simulink model "virtualPendulumModel"  (R2022a)
settings: Solver=FixedStepAuto  StartTime=0.0  StopTime=10  FixedStep=model.ts  RelTol=1e-3
InitFcn:
  | Ts = 0.01;
undefined symbols (not defined in the file): Discrete, model, Time, X, Y, Z
libraries: sm_lib x8, nesl_utility x3, simulink x2, sharedTrackingLibrary x1, ctrlSharedLib x1
settings Model: Creator=mulusoy  LastModifiedBy=gioel
settings DebuggingCC: UnconnectedInputMsg=warning  UnconnectedOutputMsg=warning  UnconnectedLineMsg=warning
settings RTWCC: DLArmComputeVersion=19.05
settings ExplorerConfigSet: InternalSimMechanicsExplorerSettings="<ExplorerConfiguration><canonicalview>planar_xy</canonicalview><AnimationSetting><BasePlaybackSpeed>1.0</BasePlaybackSpeed><PlaybackSpeedFactor>1.0</PlaybackSpeedFactor></AnimationSetting><TilePanel><TileInfo><Tiles Columns=\"1\" Count=\"1\" Rows=\"1\"><Column Weight=\"1\"/><Row Weight=\"1\"/><Tile Height=\"1\" Width=\"1\" X=\"0\" Y=\"0\"/></Tiles></TileInfo><SceneInfo><SceneViewer><BGColor><R>0.60000002384185791</R><G>0.60000002384185791</G><B>0.60000002384185791</B></BGColor><Camera><DoPerspective>off</DoPerspective><Position><X>-2.81337411700555151e-09</X><Y>-0.263610325606282447</Y><Z>1.00000001491760937</Z></Position><Center><X>-2.81337411700555151e-09</X><Y>-0.263610325606282447</Y><Z>1.49176093700020829e-08</Z></Center><Up><X>0</X><Y>1</Y><Z>0</Z></Up><ViewLimDist>1</ViewLimDist><YLim>0.297268618643283855</YLim><XLim>0.57836459223084502</XLim></Camera></SceneViewer></SceneInfo></TilePanel><MechEditorPanel><Cameras/><GfxPanelCameraMap/><VideoCreator><PlaybackSpeedRatio>1.0</PlaybackSpeedRatio><FrameRate>30</FrameRate><VideoFormat>Motion JPEG AVI</VideoFormat><FrameSize>auto</FrameSize></VideoCreator></MechEditorPanel></ExplorerConfiguration>"

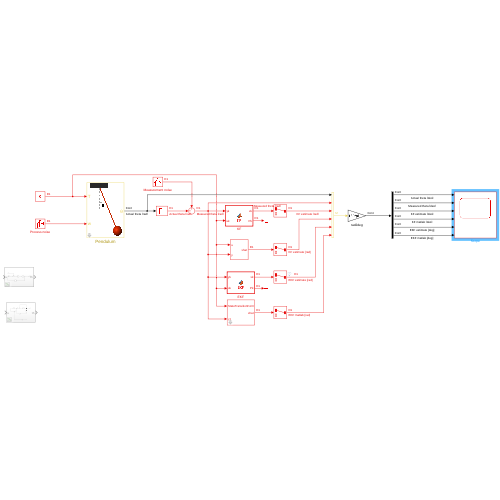
[thumbnail: Simulink's stored preview of the top-level diagram]
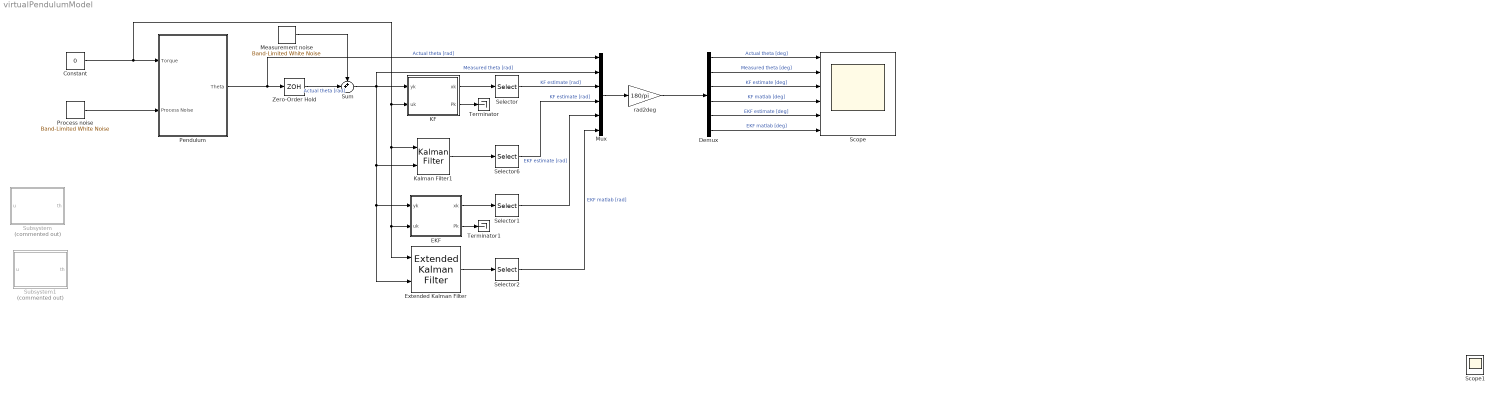
== system virtualPendulumModel ==
  Constant : Constant  Value=0  SampleTime=model.ts
  Demux : Demux  Outputs=6
  EKF : MATLAB Function  TreatAsAtomicUnit=on
  Extended Kalman Filter : sharedTrackingLibrary/Extended Kalman Filter  StateTransitionFcn=myStateTransitionFcn  HasStateTransitionJacobianFcn=off  HasAdditiveProcessNoise=Additive  ProcessNoise=model.Q  HasTimeVaryingProcessNoise=off  HasStateTransitionFcnExtraArgument=1  InitialState=[model.theta0; model.theta_dot0]  InitialStateCovariance=model.dis_lin.P0  MeasurementFcn1=myMeasurementFcn  HasMeasurementJacobianFcn1=off  HasMeasurementEnablePort1=off  HasAdditiveMeasurementNoise1=Additive  MeasurementNoise1=model.R  HasTimeVaryingMeasurementNoise1=off  HasMeasurementFcnExtraArgument1=0  HasMeasurementWrapping1=off  MeasurementFcn2=myMeasurementFcn  HasMeasurementJacobianFcn2=off  HasMeasurementEnablePort2=off  HasAdditiveMeasurementNoise2=Additive  MeasurementNoise2=1  HasTimeVaryingMeasurementNoise2=off  HasMeasurementFcnExtraArgument2=0  HasMeasurementWrapping2=off  MeasurementFcn3=myMeasurementFcn  HasMeasurementJacobianFcn3=off  HasMeasurementEnablePort3=off  HasAdditiveMeasurementNoise3=Additive  MeasurementNoise3=1  HasTimeVaryingMeasurementNoise3=off  HasMeasurementFcnExtraArgument3=0  HasMeasurementWrapping3=off  MeasurementFcn4=myMeasurementFcn  HasMeasurementJacobianFcn4=off  HasMeasurementEnablePort4=off  HasAdditiveMeasurementNoise4=Additive  MeasurementNoise4=1  HasTimeVaryingMeasurementNoise4=off  HasMeasurementFcnExtraArgument4=0  HasMeasurementWrapping4=off  MeasurementFcn5=myMeasurementFcn  HasMeasurementJacobianFcn5=off  HasMeasurementEnablePort5=off  HasAdditiveMeasurementNoise5=Additive  MeasurementNoise5=1  HasTimeVaryingMeasurementNoise5=off  HasMeasurementFcnExtraArgument5=0  HasMeasurementWrapping5=off  EnableMultirate=off  StateTransitionFcnSampleTime=1  MeasurementFcn1SampleTime=1  MeasurementFcn2SampleTime=1  MeasurementFcn3SampleTime=1  MeasurementFcn4SampleTime=1  MeasurementFcn5SampleTime=1  UseCurrentEstimator=on  OutputStateCovariance=off  DataType=double  SampleTime=model.ts  NumberOfMeasurements=1
      settings: SourceProductBaseCode=TF,AE,PW,CT,DR,ID,LP,NV,AR,RO,RR,UV,VE
  KF : MATLAB Function  TreatAsAtomicUnit=on
  Kalman Filter1 : ctrlSharedLib/Kalman Filter  TimeDomain=Discrete-Time  UseCurrentEstimator=on  ModelSource=Individual A, B, C, D matrices  ModelSourceVariable=ss(0.95,1,1,0,1)  A=model.dis_lin.A  B=model.dis_lin.B  C=model.dis_lin.C  D=model.dis_lin.D  NumberOfStates=1  NumberOfInputs=1  NumberOfOutputs=1  InitialEstimateSource=Dialog  X0=[model.theta0; model.theta_dot0]  P0=10  UseK=off  UseGH=off  NumberOfProcessNoiseInputs=1  G=1  TimeInvariantG=on  H=0  TimeInvariantH=on  Q=model.Q  TimeInvariantQ=on  R=model.R  TimeInvariantR=on  N=0  TimeInvariantN=on  AddInputPort=on  AddEnablePort=off  OutputEstimatedY=off  OutputP=off  Ts=model.ts
  Measurement noise : simulink/Sources/Band-Limited White Noise  Cov=model.R*model.ts  Ts=model.ts  seed=[23341]
  Mux : Mux  Inputs=6
  Pendulum : Subsystem  mask{theta_0=model.theta0, theta_dot_0=model.theta_dot0}
      mask prompts: theta_0 "Initial value of theta"; theta_dot_0 "Initial value of theta_dot"
      mask Display:
      | image('pend.png');
      | port_label('input',1,'T');
      | port_label('input',2,'w');
      | port_label('output',1,'\theta','interpreter','tex');
  Process noise : simulink/Sources/Band-Limited White Noise  Cov=model.Q(2,2)*model.ts  Ts=model.ts  seed=[23341]
  Scope : Scope  NumInputPorts=6
  Selector{,1..2,6} (4 alike) : Selector  InputPortWidth=2  IndexOptions=Index vector (dialog)  Indices=[1]  OutputSizes=1
  Subsystem : Subsystem  Commented=on
  Subsystem1 : Subsystem  Commented=on
  Sum : Sum  Inputs=++|
  Terminator : Terminator
  Terminator1 : Terminator
  Zero-Order Hold : ZeroOrderHold  SampleTime=model.ts
  rad2deg : Gain  Gain=180/pi
  Scope1 : Scope
  wires:
  Measurement noise/1 -> Sum/1
  Process noise/1 -> Pendulum/2(Process Noise)
  KF/1(xk) -> Selector/1
  Selector/1 -> Mux/3  "KF estimate [rad]"
  Mux/1 -> rad2deg/1
  KF/2(Pk) -> Terminator/1
  Sum/1 -> Extended Kalman Filter/2, EKF/1(yk), Kalman Filter1/2, Mux/2, KF/1(yk)  "Measured theta [rad]"
  Zero-Order Hold/1 -> Sum/2  "Actual theta [rad]"
  Pendulum/1(Theta) -> Mux/1, Zero-Order Hold/1  "Actual theta [rad]"
  EKF/2(Pk) -> Terminator1/1
  EKF/1(xk) -> Selector1/1
  Selector1/1 -> Mux/5  "EKF estimate [rad]"
  Constant/1 -> EKF/2(uk), Extended Kalman Filter/1, Kalman Filter1/1, KF/2(uk), Pendulum/1(Torque)
  Extended Kalman Filter/1 -> Selector2/1
  Selector2/1 -> Mux/6  "EKF matlab [rad]"
  Kalman Filter1/1 -> Selector6/1
  Demux/6 -> Scope/6  "EKF matlab [deg]"
  Demux/5 -> Scope/5  "EKF estimate [deg]"
  Demux/3 -> Scope/3  "KF estimate [deg]"
  Demux/2 -> Scope/2  "Measured theta [deg]"
  Demux/1 -> Scope/1  "Actual theta [deg]"
  rad2deg/1 -> Demux/1
  Selector6/1 -> Mux/4  "KF estimate [rad]"
  Demux/4 -> Scope/4  "KF matlab [deg]"

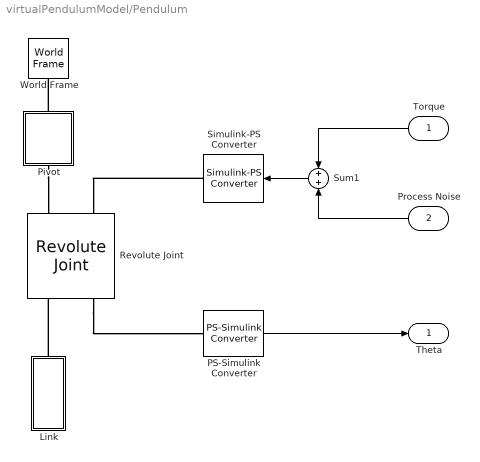
== system virtualPendulumModel/Pendulum ==
  Torque : Inport
  Process Noise : Inport  Port=2
  Link : Subsystem  Tag=CustomStyle
  PS-Simulink Converter : nesl_utility/PS-Simulink Converter  PhysicalDomain=network_engine_domain  SubClassName=ps_output  LeftPortType=input  RightPortType=output  PseudoPeriodic=off  Frequencies=[]  VectorFormat=1-D array  Unit=1  AffineConversion=off
      settings: SourceProductBaseCode=SS,PW,VE
  Pivot : Subsystem  Tag=CustomStyle
  Revolute Joint : sm_lib/Joints/Revolute Joint  JointMode=Normal  SenseConstraintForce=off  SenseConstraintForceX=off  SenseConstraintForceY=off  SenseConstraintForceZ=off  SenseConstraintTorque=off  SenseConstraintTorqueX=off  SenseConstraintTorqueY=off  SenseConstraintTorqueZ=off  SenseTotalForce=off  SenseTotalForceX=off  SenseTotalForceY=off  SenseTotalForceZ=off  SenseTotalTorque=off  SenseTotalTorqueX=off  SenseTotalTorqueY=off  SenseTotalTorqueZ=off  CompositeWrenchDir=FollowerOnBase  CompositeWrenchFrame=BaseFrame  EquilibriumPosition=0  EquilibriumPositionUnits=rad  SpringStiffness=0  SpringStiffnessUnits=N*m/rad  DampingCoefficient=0  DampingCoefficientUnits=N*m/(rad/s)  TorqueActuationMode=InputTorque  MotionActuationMode=ComputedMotion  SensePosition=on  SenseVelocity=off  SenseAcceleration=off  SenseTorqueForce=off  SenseLowerLimitTorqueForce=off  SenseUpperLimitTorqueForce=off  LowerLimitSpecify=off  LowerLimitBound=-90  LowerLimitBoundUnits=deg  LowerLimitStiffness=1e4  LowerLimitStiffnessUnits=N*m/deg  LowerLimitDamping=10  LowerLimitDampingUnits=N*m/(deg/s)  LowerLimitTransitionRegionWidth=0.1  LowerLimitTransitionRegionWidthUnits=deg  UpperLimitSpecify=off  UpperLimitBound=90  UpperLimitBoundUnits=deg  UpperLimitStiffness=1e4  UpperLimitStiffnessUnits=N*m/deg  UpperLimitDamping=10  UpperLimitDampingUnits=N*m/(deg/s)  UpperLimitTransitionRegionWidth=0.1  UpperLimitTransitionRegionWidthUnits=deg  PositionTargetSpecify=on  PositionTargetPriority=High  PositionTargetValue=model.theta0  PositionTargetValueUnits=rad  VelocityTargetSpecify=on  VelocityTargetPriority=High  VelocityTargetValue=model.theta_dot0  VelocityTargetValueUnits=rad/s
  Simulink-PS Converter : nesl_utility/Simulink-PS Converter  PhysicalDomain=network_engine_domain  SubClassName=ps_input  LeftPortType=input  RightPortType=output  PseudoPeriodic=off  Frequencies=[]  NoiseDistribution=none  NoiseParameters=[]  Unit=1  AffineConversion=off  FilteringAndDerivatives=provide  SimscapeFilterOrder=1  InputFilterTimeConstant=0.001  UdotUserProvided=0
      settings: SourceProductBaseCode=SS,PW,VE
  Sum1 : Sum  Inputs=+|+
  World Frame : sm_lib/Frames and Transforms/World Frame
  Theta : Outport
  wires:
  Sum1/1 -> Simulink-PS Converter/1
  Torque/1 -> Sum1/1
  Process Noise/1 -> Sum1/2
  PS-Simulink Converter/1 -> Theta/1
  connections:
  Pivot/LConn1 -- World Frame/RConn1
  Pivot/RConn1 -- Revolute Joint/LConn1
  Link/RConn1 -- Revolute Joint/RConn1
  Revolute Joint/RConn2 -- PS-Simulink Converter/LConn1
  Simulink-PS Converter/RConn1 -- Revolute Joint/LConn2

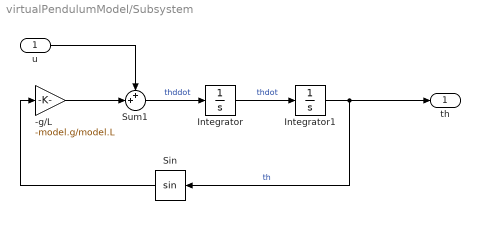
== system virtualPendulumModel/Subsystem ==
  u : Inport
  -g/L : Gain  Gain=-model.g/model.L
  Integrator : Integrator  InitialCondition=model.theta_dot0
  Integrator1 : Integrator  InitialCondition=model.theta0
  Sin : Trigonometry
  Sum1 : Sum  Inputs=++|
  th : Outport
  wires:
  Sum1/1 -> Integrator/1  "thddot"
  Integrator/1 -> Integrator1/1  "thdot"
  Sin/1 -> -g/L/1
  u/1 -> Sum1/1
  Integrator1/1 -> th/1, Sin/1  "th"
  -g/L/1 -> Sum1/2

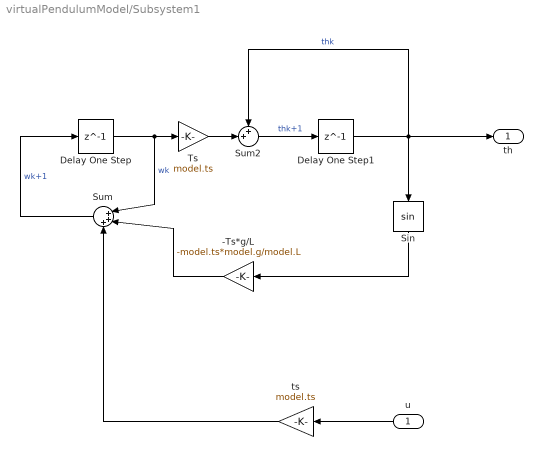
== system virtualPendulumModel/Subsystem1 ==
  u : Inport
  -Ts*g/L : Gain  Gain=-model.ts*model.g/model.L
  Delay One Step : Delay  DelayLength=1  InitialCondition=model.theta_dot0
  Delay One Step1 : Delay  DelayLength=1  InitialCondition=model.theta0
  Sin : Trigonometry
  Sum : Sum  Inputs=|+++
  Sum2 : Sum  Inputs=++|
  Ts : Gain  Gain=model.ts
  ts : Gain  Gain=model.ts
  th : Outport
  wires:
  -Ts*g/L/1 -> Sum/2
  ts/1 -> Sum/3
  u/1 -> ts/1
  Sin/1 -> -Ts*g/L/1
  Delay One Step/1 -> Sum/1, Ts/1  "wk"
  Ts/1 -> Sum2/2
  Sum2/1 -> Delay One Step1/1  "thk+1"
  Delay One Step1/1 -> th/1, Sin/1, Sum2/1  "thk"
  Sum/1 -> Delay One Step/1  "wk+1"

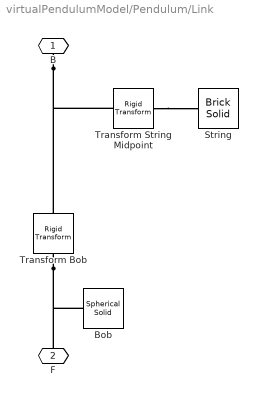
== system virtualPendulumModel/Pendulum/Link ==
  Bob : sm_lib/Body Elements/Spherical Solid  GraphicAmbientColor=[0.15 0.15 0.15 1.0]  BasedOnType=Density  CenterOfMass=[0 0 0]  CenterOfMassUnits=m  GraphicDiffuseColor=[1.0 0.2 0.0]  Density=1000  DensityUnits=kg/(m^3)  DoExposeReferenceFrame=on  GraphicEmissiveColor=[0.0 0.0 0.0 1.0]  ExportEntireGeometry=off  SerializedExposedGeometries=<ExposedGeometries/>  SerializedFrames=<Frames/>  MarkerShape=Sphere  MarkerSize=10  GraphicType=FromGeometry  InertiaType=PointMass  Mass=model.m  MassUnits=kg  MomentsOfInertia=[1 1 1]*1e-3  MomentsOfInertiaUnits=kg*m^2  GraphicOpacity=1.0  ProductsOfInertia=[0 0 0]  ProductsOfInertiaUnits=kg*m^2  GraphicShininess=75  GraphicSpecularColor=[0.5 0.5 0.5 1.0]  SphereRadius=0.05  SphereRadiusUnits=m  GraphicVisPropType=SimpleVisualProperties
  String : sm_lib/Body Elements/Brick Solid  GraphicAmbientColor=[0.15 0.15 0.15 1.0]  BasedOnType=Density  BrickDimensions=[0.01 model.L 0.01]  BrickDimensionUnits=m  CenterOfMass=[0 0 0]  CenterOfMassUnits=m  GraphicDiffuseColor=[1.0 0.2 0.0]  Density=0  DensityUnits=kg/(m^3)  DoExposeReferenceFrame=on  GraphicEmissiveColor=[0.0 0.0 0.0 1.0]  ExportEntireGeometry=off  SerializedFrames=<Frames/>  MarkerShape=Sphere  MarkerSize=10  GraphicType=FromGeometry  InertiaType=CalculateFromGeometry  Mass=0  MassUnits=kg  MomentsOfInertia=[1 1 1]*1e-3  MomentsOfInertiaUnits=kg*m^2  GraphicOpacity=1.0  ProductsOfInertia=[0 0 0]  ProductsOfInertiaUnits=kg*m^2  GraphicShininess=75  GraphicSpecularColor=[0.5 0.5 0.5 1.0]  GraphicVisPropType=SimpleVisualProperties
  "Transform Bob " : sm_lib/Frames and Transforms/Rigid Transform  TranslationMethod=StandardAxis  TranslationStandardOffset=model.L  TranslationLengthUnit=m  TranslationStandardAxis=-Y  TranslationCartesianOffset=[0 0 0]  TranslationROffset=0  TranslationROffsetUnits=m  TranslationZOffset=0  TranslationZOffsetUnits=m  TranslationThetaOffset=0  TranslationThetaOffsetUnits=deg  RotationMethod=None  RotationAngleUnits=deg  RotationStandardAxis=+Z  RotationAngle=0  RotationArbitraryAxis=[0 0 1]  FollAlignAxisA=+X  BaseAlignAxisA=+Y  FollAlignAxisB=+Y  BaseAlignAxisB=+Z  RotationSequenceAxes=FollowerAxes  RotationSequence=XYX  RotationSequenceAngles=[0 0 0]  RotationSequenceAnglesUnits=deg  RotationMatrix=[1 0 0; 0 1 0; 0 0 1]
  Transform String Midpoint : sm_lib/Frames and Transforms/Rigid Transform  TranslationMethod=StandardAxis  TranslationStandardOffset=model.L/2  TranslationLengthUnit=m  TranslationStandardAxis=-Y  TranslationCartesianOffset=[0 0 0]  TranslationROffset=0  TranslationROffsetUnits=m  TranslationZOffset=0  TranslationZOffsetUnits=m  TranslationThetaOffset=0  TranslationThetaOffsetUnits=deg  RotationMethod=None  RotationAngleUnits=deg  RotationStandardAxis=+Z  RotationAngle=0  RotationArbitraryAxis=[0 0 1]  FollAlignAxisA=+X  BaseAlignAxisA=+Y  FollAlignAxisB=+Y  BaseAlignAxisB=+Z  RotationSequenceAxes=FollowerAxes  RotationSequence=XYX  RotationSequenceAngles=[0 0 0]  RotationSequenceAnglesUnits=deg  RotationMatrix=[1 0 0; 0 1 0; 0 0 1]
  B : PMIOPort  Side=Right
  F : PMIOPort  Port=2  Side=Left
  connections:
  Transform String Midpoint/RConn1 -- String/RConn1
  "Transform Bob "/RConn1 -- F/RConn1 -- Bob/RConn1
  B/RConn1 -- Transform String Midpoint/LConn1 -- "Transform Bob "/LConn1

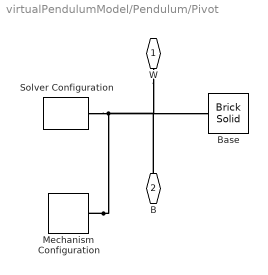
== system virtualPendulumModel/Pendulum/Pivot ==
  Base : sm_lib/Body Elements/Brick Solid  GraphicAmbientColor=[0.15 0.15 0.15 1.0]  BasedOnType=Density  BrickDimensions=[0.2 0.05 0.1]  BrickDimensionUnits=m  CenterOfMass=[0 0 0]  CenterOfMassUnits=m  GraphicDiffuseColor=[0.2 0.2 0.2]  Density=1000  DensityUnits=kg/(m^3)  DoExposeReferenceFrame=on  GraphicEmissiveColor=[0.0 0.0 0.0 1.0]  ExportEntireGeometry=off  SerializedFrames=<Frames/>  MarkerShape=Sphere  MarkerSize=10  GraphicType=FromGeometry  InertiaType=CalculateFromGeometry  Mass=1  MassUnits=kg  MomentsOfInertia=[1 1 1]*1e-3  MomentsOfInertiaUnits=kg*m^2  GraphicOpacity=1.0  ProductsOfInertia=[0 0 0]  ProductsOfInertiaUnits=kg*m^2  GraphicShininess=75  GraphicSpecularColor=[0.5 0.5 0.5 1.0]  GraphicVisPropType=SimpleVisualProperties
  Mechanism Configuration : sm_lib/Utilities/Mechanism Configuration  UniformGravity=Constant  GravityVector=[0 -model.g 0]  GravityUnits=m/s^2  LinearizationDelta=0.001  JointModeTransitionNonlinearIterations=2
  Solver Configuration : nesl_utility/Solver Configuration  PhysicalDomain=network_engine_domain  SubClassName=solver  LeftPortType=input  RightPortType=generic  Tones=[]  Harmonics=[]  SimulateNoise=off  Profile=off  UseLocalSampling=off  EnableSwitchedLinearOptims=on  FrequencyDomain=off  UseCCode=off  RelTol=0.001  AbsTol=1e-06  MinStep=1e-09  ToWorkspace=off  RevertToSquareIcSolve=off  NumHomotopyIterations=100  PhasorMode=off  PhasorModeNumHarmonics=1  IndexReductionMethod=DerivativeReplacement  DoDC=off  ResidualTolerance=1e-9  UseLocalSolver=off  LocalSolverChoice=NE_BACKWARD_EULER_ADVANCER  LocalSolverSampleTime=.001  DoFixedCost=off  MaxNonlinIter=3  MaxModeIter=2  ComputeImpulses=off  ImpulseIterations=2  LinearAlgebra=Sparse  LinearAlgebraNumThread=0  EquationFormulation=NE_TIME_EF  DelaysMemoryBudget=1024  AutomaticFiltering=on  FilteringTimeConstant=0.001  PartitionStorageMethod=AS_NEEDED  PartitionMemoryBudget=1024  PartitionMethod=FAST
      settings: SourceProductBaseCode=SS,PW,VE
  W : PMIOPort  Side=Left
  B : PMIOPort  Port=2  Side=Right
  connections:
  Mechanism Configuration/RConn1 -- Solver Configuration/RConn1 -- B/RConn1 -- Base/RConn1 -- W/RConn1

== matlab function virtualPendulumModel/KF ==
  data: yk input; uk input; xk output; model parameter; Pk output
function [xk,Pk] = KF(yk, uk, model)

% Persistent variables which take into account previous 
% state-covariance estimates
persistent xk_1;
persistent Pk_1;

if isempty(xk_1)

    % Initialize state estimate and covariance estimate
    xk_1 = model.dis_lin.x0est;
    Pk_1 = model.dis_lin.P0;
    xk = xk_1;
    Pk = Pk_1;

else

    % Prediction step
    xk_ = model.dis_lin.A * xk_1 + model.dis_lin.B * uk;
    Pk_ = model.dis_lin.A * Pk_1 * transpose(model.dis_lin.A) + model.Q;
    
    % Update step
    Kk = Pk_ * transpose(model.dis_lin.C) / (model.dis_lin.C * Pk_ * transpose(model.dis_lin.C) + model.R);
    xk = xk_ + Kk * (yk - model.dis_lin.C * xk_);
    xk_1 = xk;
    Pk = (eye(size(xk_,1)) - Kk * model.dis_lin.C) * Pk_;
    Pk_1 = Pk;

end

== matlab function virtualPendulumModel/EKF ==
  data: yk input; uk input; xk output; model parameter; Pk output
function [xk, Pk] = EKF(yk, uk, model)

% Persistent variables which take into account previous 
% state-covariance estimates
persistent xke_1;
persistent Pke_1;

if isempty(xke_1)

    % Initialize state estimate and covariance estimate
    xke_1 = model.dis_lin.x0est;
    Pke_1 = model.dis_lin.P0;
    xk = xke_1;
    Pk = Pke_1;

else

    % Compute jacobians
    A = [model.dis_lin.A(1,1) model.dis_lin.A(1,2);
         -model.dis_lin.A(2,1)*cos(xke_1(1)) model.dis_lin.A(2,2)];
    C = [1 0];

    % Prediction step
    xk_ = [xke_1(1) + model.ts*xke_1(2);
           xke_1(2) + model.dis_lin.A(2,1)*sin(xke_1(1))] + model.dis_lin.B * uk;
    Pk_ = A * Pke_1 * transpose(A) + model.Q;
  
    % Update step
    Kk = Pk_ * transpose(C) / (C * Pk_ * transpose(C) + model.R);
    xk = xk_ + Kk * (yk - C * xk_);
    Pk = (eye(size(xk_,1)) - Kk * C) * Pk_ * transpose(eye(size(xk_,1)) - Kk * C) + Kk * model.R * transpose(Kk);
    xke_1 = xk;
    Pke_1 = Pk;
end
